simulink model "SystemDiagram"  (R2024a)
settings: Solver=VariableStepAuto  StartTime=0.0  StopTime=4  RelTol=1e-3
undefined symbols (not defined in the file): A, B, k
settings Model: Creator=alhjkadouro  LastModifiedBy=alhjkadouro
settings DataIOCC: ExternalInput=controller

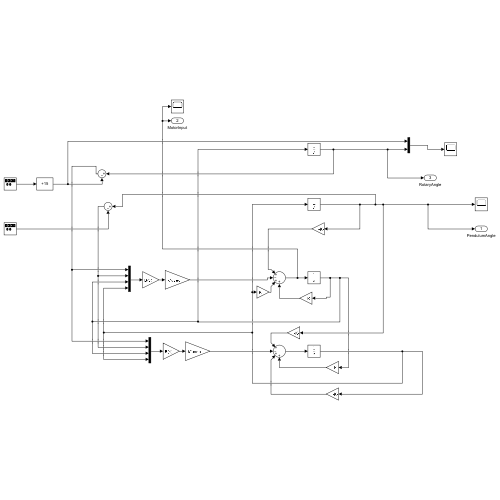
[thumbnail: Simulink's stored preview of the top-level diagram]
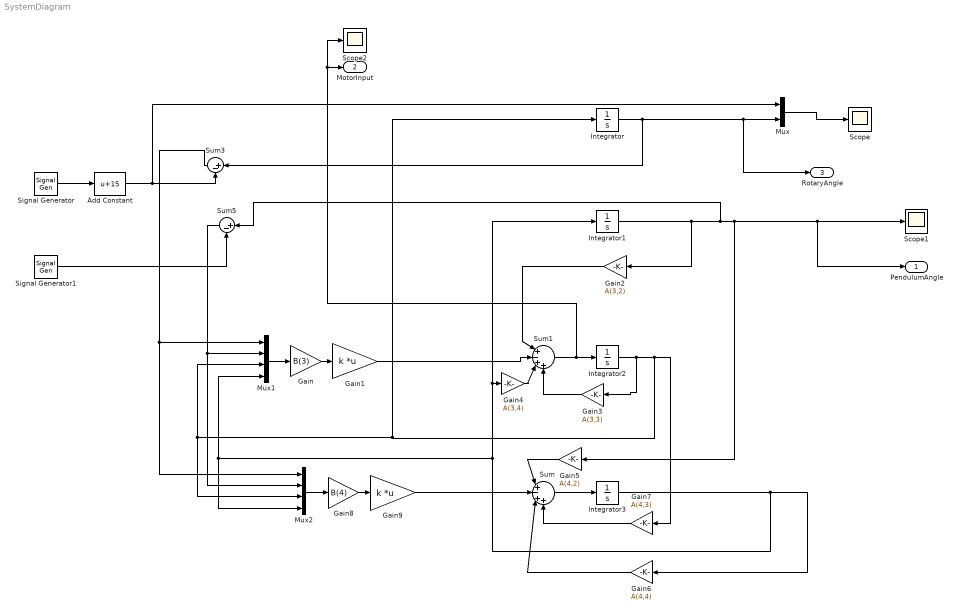
== system SystemDiagram ==
  Add Constant : Bias  Bias=15  SaturateOnIntegerOverflow=off
  Gain : Gain  Gain=B(3)
  Gain1 : Gain  Gain=k  Multiplication=Matrix(K*u) (u vector)
  Gain2 : Gain  Gain=A(3,2)
  Gain3 : Gain  Gain=A(3,3)
  Gain4 : Gain  Gain=A(3,4)
  Gain5 : Gain  Gain=A(4,2)
  Gain6 : Gain  Gain=A(4,4)
  Gain7 : Gain  Gain=A(4,3)
  Gain8 : Gain  Gain=B(4)
  Gain9 : Gain  Gain=k  Multiplication=Matrix(K*u) (u vector)
  Integrator{,1..3} (4 alike) : Integrator
  Mux : Mux  Inputs=2
  Mux1 : Mux
  Mux2 : Mux
  Scope : Scope
  Scope1 : Scope
  Scope2 : Scope
  Signal Generator : SignalGenerator  WaveForm=square  Amplitude=-15  Frequency=0.1
  Signal Generator1 : SignalGenerator  WaveForm=square  Amplitude=0  Frequency=0.125
  Sum : Sum  Inputs=|+-++
  Sum1 : Sum  Inputs=|+-++
  Sum3 : Sum  Inputs=|+-
  Sum5 : Sum  Inputs=|+-
  PendulumAngle : Outport
  MotorInput : Outport  Port=2
  RotaryAngle : Outport  Port=3
  wires:
  Sum1/1 -> Scope2/1, MotorInput/1, Integrator2/1
  Sum/1 -> Integrator3/1
  Gain2/1 -> Sum1/1
  Gain3/1 -> Sum1/4
  Gain4/1 -> Sum1/3
  Integrator/1 -> Sum3/1, RotaryAngle/1, Mux/2
  Gain5/1 -> Sum/1
  Gain7/1 -> Sum/4
  Gain6/1 -> Sum/3
  Integrator2/1 -> Gain7/1, Mux2/3, Mux1/3, Integrator/1, Gain3/1
  Integrator3/1 -> Mux2/4, Mux1/4, Gain4/1, Integrator1/1, Gain6/1
  Integrator1/1 -> Sum5/1, PendulumAngle/1, Scope1/1, Gain5/1, Gain2/1
  Gain9/1 -> Sum/2
  Sum3/1 -> Mux2/1, Mux1/1
  Signal Generator/1 -> Add Constant/1
  Sum5/1 -> Mux2/2, Mux1/2
  Signal Generator1/1 -> Sum5/2
  Mux/1 -> Scope/1
  Add Constant/1 -> Mux/1, Sum3/2
  Mux1/1 -> Gain/1
  Gain/1 -> Gain1/1
  Mux2/1 -> Gain8/1
  Gain8/1 -> Gain9/1
  Gain1/1 -> Sum1/2
